simulink model "Klimaanlage_SIL"  (R2023b)
settings: Solver=FixedStepAuto  StartTime=0.0  StopTime=10.0  RelTol=1e-3
values from neighbouring files (symbols this model uses):
  T_a = 5    [qualification_test_01.m]    (also in qualification_test_02.m)
  T_i_start = 10    [qualification_test_01.m]    (also in qualification_test_02.m)
libraries: mbedblockslib x10, thermical_vehicelbody x1
settings Model: Creator=kilia  LastModifiedBy=kilia
settings HardwareCC: TargetBitPerPointer=64  TargetBitPerSizeT=64  TargetBitPerPtrDiffT=64  TargetLongLongMode=on  TargetIntDivRoundTo=Zero  TargetEndianess=LittleEndian  TargetWordSize=64  TargetHWDeviceType=MATLAB Host  ProdEqTarget=off
settings RTWCC: Description=S-Function Target  SystemTargetFile=rtwsfcn.tlc  TemplateMakefile=rtwsfcn_default_tmf
settings STFCustomTargetCC: ModelReferenceCompliant=off  CompOptLevelCompliant=on  MATLABClassNameForMDSCustomization=Simulink.SoftwareTarget.TargetSpecificTriggerConfigurationBase  GRTInterface=on  SystemTargetFile=rtwsfcn.tlc

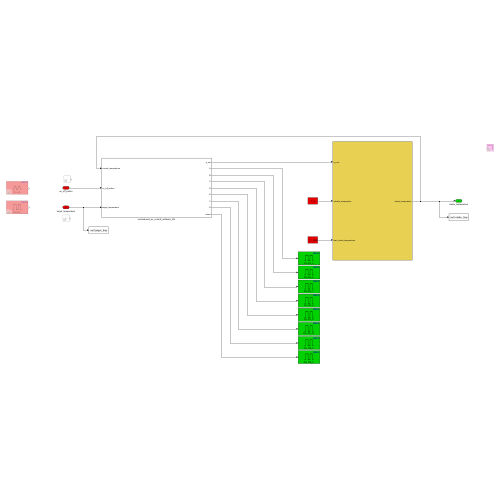
[thumbnail: Simulink's stored preview of the top-level diagram]
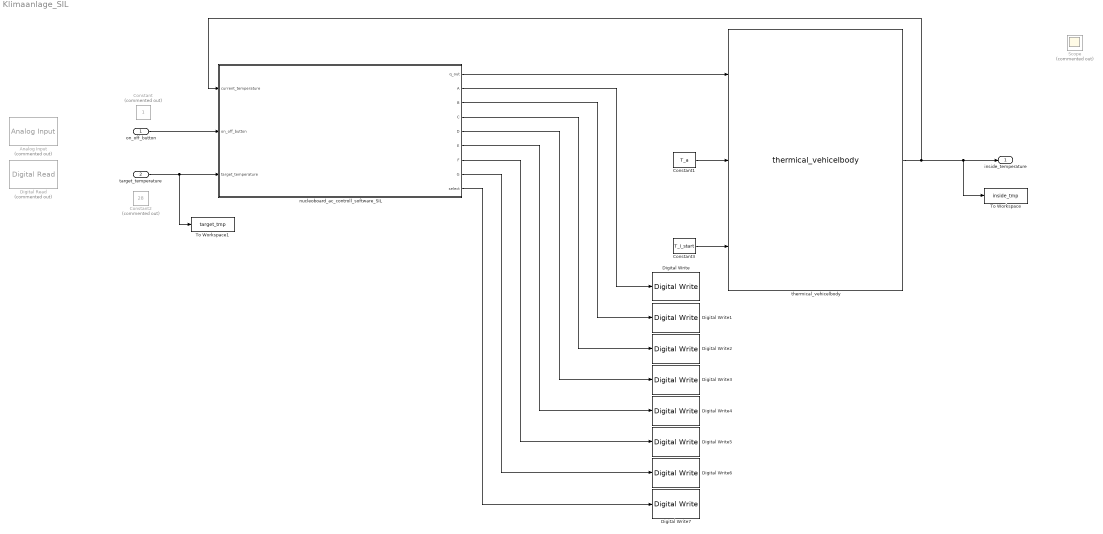
== system Klimaanlage_SIL ==
  on_off_button : Inport  OutDataTypeStr=boolean
  target_temperature : Inport  Port=2
  Analog Input : mbedblockslib/Analog Input  Commented=on  Pin=A0  ReadResultsOnly=off  ConversionTriggerSource=Software  ExternalTriggerType=uint32( 0 )  OutputDataType=double  EnableConversionCompleteNotify=off  EnableOuputStatus=off  SampleTime=-1
      settings: LibrarySourceBlock=stmnucleorootlib/Common/Analog Input
  Constant : Constant  Commented=on  OutDataTypeStr=boolean
  Constant1 : Constant  Value=T_a
  Constant2 : Constant  Commented=on  Value=28  OutDataTypeStr=uint16
  Constant3 : Constant  Value=T_i_start
  Digital Read : mbedblockslib/Digital Read  Commented=on  Pin=D2  Direction=input  SampleTime=-1
      settings: LibrarySourceBlock=stmnucleorootlib/Common/Digital Read
  Digital Write : mbedblockslib/Digital Write  Pin=PA_5  Direction=output
      settings: LibrarySourceBlock=stmnucleorootlib/Common/Digital Write
  Digital Write1 : mbedblockslib/Digital Write  Pin=PA_6  Direction=output
      settings: LibrarySourceBlock=stmnucleorootlib/Common/Digital Write
  Digital Write2 : mbedblockslib/Digital Write  Pin=PA_7  Direction=output
      settings: LibrarySourceBlock=stmnucleorootlib/Common/Digital Write
  Digital Write3 : mbedblockslib/Digital Write  Pin=PA_8  Direction=output
      settings: LibrarySourceBlock=stmnucleorootlib/Common/Digital Write
  Digital Write4 : mbedblockslib/Digital Write  Pin=PA_9  Direction=output
      settings: LibrarySourceBlock=stmnucleorootlib/Common/Digital Write
  Digital Write5 : mbedblockslib/Digital Write  Pin=PA_15  Direction=output
      settings: LibrarySourceBlock=stmnucleorootlib/Common/Digital Write
  Digital Write6 : mbedblockslib/Digital Write  Pin=PB_9  Direction=output
      settings: LibrarySourceBlock=stmnucleorootlib/Common/Digital Write
  Digital Write7 : mbedblockslib/Digital Write  Pin=PB_0  Direction=output
      settings: LibrarySourceBlock=stmnucleorootlib/Common/Digital Write
  Scope : Scope  Commented=on
  To Workspace : ToWorkspace  VariableName=inside_tmp  SaveFormat=Timeseries  SampleTime=-1
  To Workspace1 : ToWorkspace  VariableName=target_tmp  SaveFormat=Timeseries  SampleTime=-1
  nucleoboard_ac_controll_software_SIL : Subsystem
      mask help: Simulink:masks:GenSFuncDesc_MD
      mask Help: eval('feval(''rtwprivate'',''rtwhelpview'',''rtw_sfcn_block'')');
  thermical_vehicelbody : thermical_vehicelbody/thermical_vehicelbody  SystemSampleTime=-1  VariantActivationTime=update diagram  AllowFlexibleInterface=on  Latency=0  AutoFrameSizeCalculation=off
  inside_temperature : Outport
  wires:
  nucleoboard_ac_controll_software_SIL/8(G) -> Digital Write6/1
  nucleoboard_ac_controll_software_SIL/9(select) -> Digital Write7/1
  nucleoboard_ac_controll_software_SIL/6(E) -> Digital Write4/1
  Constant3/1 -> thermical_vehicelbody/3
  nucleoboard_ac_controll_software_SIL/3(B) -> Digital Write1/1
  nucleoboard_ac_controll_software_SIL/4(C) -> Digital Write2/1
  nucleoboard_ac_controll_software_SIL/7(F) -> Digital Write5/1
  nucleoboard_ac_controll_software_SIL/2(A) -> Digital Write/1
  nucleoboard_ac_controll_software_SIL/1(q_out) -> thermical_vehicelbody/1
  thermical_vehicelbody/1 -> To Workspace/1, inside_temperature/1, nucleoboard_ac_controll_software_SIL/1(current_temperature)
  Constant1/1 -> thermical_vehicelbody/2
  target_temperature/1 -> To Workspace1/1, nucleoboard_ac_controll_software_SIL/3(target_temperature)
  on_off_button/1 -> nucleoboard_ac_controll_software_SIL/2(on_off_button)
  nucleoboard_ac_controll_software_SIL/5(D) -> Digital Write3/1

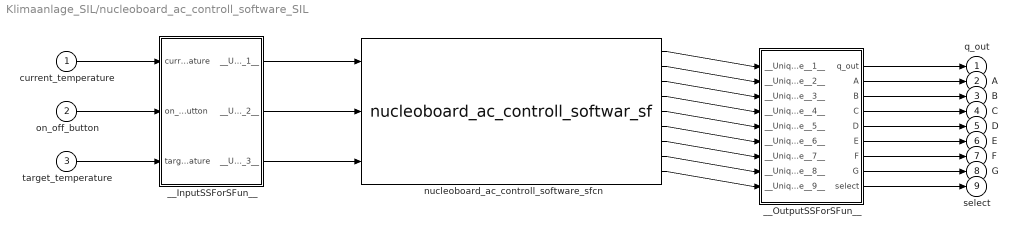
== system Klimaanlage_SIL/nucleoboard_ac_controll_software_SIL ==
  current_temperature : Inport
  on_off_button : Inport  Port=2
  target_temperature : Inport  Port=3
  __InputSSForSFun__ : Subsystem
  __OutputSSForSFun__ : Subsystem
  nucleoboard_ac_controll_software_sfcn : S-Function  FunctionName=nucleoboard_ac_controll_softwar_sf  SFunctionModules=""  SFunctionDeploymentMode=off  EnableBusSupport=off  SFcnStateName=DWORK0  mask{rtw_sf_name=nucleoboard_ac_controll_softwar_sf, showVar=off}
      mask prompts: rtw_sf_name "Simulink:masks:GenSFuncName_MP"; showVar "Simulink:masks:GenSFuncShowModuleList_MP"
      mask help: Simulink:masks:GenSFuncDesc_MD
      mask init:
      | displist = '';
      | if ~strcmp(get_param(gcb, 'FunctionName'), rtw_sf_name);
      |   set_param(gcb, 'FunctionName', rtw_sf_name);
      | end
      | % Check if we are generating code
      | rtw_mode = false;
      | if strcmpi(get_param(bdroot(gcb),'SimulationStatus'),'Initializing')
      | 	rtw_mode = strcmpi(get_param(bdroot(gcb),'BuildingRTWCode'),'on') && ...
      | 		~strcmpi(get_param(bdroot(gcb),'TargetStyle'),'SimulationTarget');
      | end
      | if showVar || rtw_mode
      | 	if exist('rtwsfunc') == 2 | exist('rtwsfunc') == 6
      | 		tmplist = rtwsfunc(rtw_sf_name,gcb);
      | 		tmplist = DAStudio.message('Simulink:masks:GenSFuncListOfModules_IC', tmplist);
      | 	elseif showVar
      | 		tmplist1 = DAStudio.message('Simulink:masks:GenSFuncListOfModules_IC', '');
      |         tmplist2 = DAStudio.message('Simulink:masks:GenSFuncNotLicensed_IC');
      |         tmplist = [tmplist1 tmplist2];
      |  	end
      | end
      | if showVar
      |   displist = tmplist;
      | end
      settings: SFcnIsStateOwnerBlock=on
      settings: CopyFcn=|
      | if ~strcmp(get_param(gcb,'Linkstatus'),'none') && ...
      | ~strcmp(get_param(gcb,'Linkstatus'),'implicit')
      |   set_param(gcb,'LinkStatus','none');
      | end
      mask Help: eval('feval(''rtwprivate'',''rtwhelpview'',''rtw_sfcn_block'')');
      mask Display:
      | port_label('input',1,'current_temperature');
      | port_label('input',2,'on_off_button');
      | port_label('input',3,'target_temperature');
      | port_label('output',1,'q_out');
      | port_label('output',2,'A');
      | port_label('output',3,'B');
      | port_label('output',4,'C');
      | port_label('output',5,'D');
      | port_label('output',6,'E');
      | port_label('output',7,'F');
      | port_label('output',8,'G');
      | port_label('output',9,'select');
  q_out : Outport
  A : Outport  Port=2
  B : Outport  Port=3
  C : Outport  Port=4
  D : Outport  Port=5
  E : Outport  Port=6
  F : Outport  Port=7
  G : Outport  Port=8
  select : Outport  Port=9
  wires:
  __OutputSSForSFun__/9(select) -> select/1
  __OutputSSForSFun__/8(G) -> G/1
  __OutputSSForSFun__/7(F) -> F/1
  __OutputSSForSFun__/6(E) -> E/1
  __OutputSSForSFun__/5(D) -> D/1
  __OutputSSForSFun__/4(C) -> C/1
  __OutputSSForSFun__/3(B) -> B/1
  __OutputSSForSFun__/2(A) -> A/1
  __OutputSSForSFun__/1(q_out) -> q_out/1
  nucleoboard_ac_controll_software_sfcn/9 -> __OutputSSForSFun__/9(__UniqueInportName__9__)
  nucleoboard_ac_controll_software_sfcn/8 -> __OutputSSForSFun__/8(__UniqueInportName__8__)
  nucleoboard_ac_controll_software_sfcn/7 -> __OutputSSForSFun__/7(__UniqueInportName__7__)
  nucleoboard_ac_controll_software_sfcn/6 -> __OutputSSForSFun__/6(__UniqueInportName__6__)
  nucleoboard_ac_controll_software_sfcn/5 -> __OutputSSForSFun__/5(__UniqueInportName__5__)
  nucleoboard_ac_controll_software_sfcn/4 -> __OutputSSForSFun__/4(__UniqueInportName__4__)
  nucleoboard_ac_controll_software_sfcn/3 -> __OutputSSForSFun__/3(__UniqueInportName__3__)
  nucleoboard_ac_controll_software_sfcn/2 -> __OutputSSForSFun__/2(__UniqueInportName__2__)
  nucleoboard_ac_controll_software_sfcn/1 -> __OutputSSForSFun__/1(__UniqueInportName__1__)
  __InputSSForSFun__/3(__UniqueOutportName__3__) -> nucleoboard_ac_controll_software_sfcn/3
  __InputSSForSFun__/2(__UniqueOutportName__2__) -> nucleoboard_ac_controll_software_sfcn/2
  __InputSSForSFun__/1(__UniqueOutportName__1__) -> nucleoboard_ac_controll_software_sfcn/1
  target_temperature/1 -> __InputSSForSFun__/3(target_temperature)
  on_off_button/1 -> __InputSSForSFun__/2(on_off_button)
  current_temperature/1 -> __InputSSForSFun__/1(current_temperature)

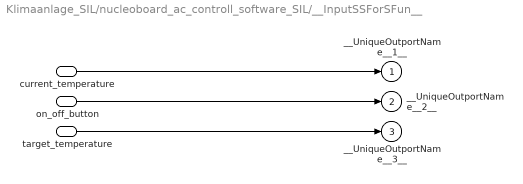
== system Klimaanlage_SIL/nucleoboard_ac_controll_software_SIL/__InputSSForSFun__ ==
  current_temperature : Inport
  on_off_button : Inport  Port=2
  target_temperature : Inport  Port=3
  __UniqueOutportName__1__ : Outport
  __UniqueOutportName__2__ : Outport  Port=2
  __UniqueOutportName__3__ : Outport  Port=3
  wires:
  target_temperature/1 -> __UniqueOutportName__3__/1
  on_off_button/1 -> __UniqueOutportName__2__/1
  current_temperature/1 -> __UniqueOutportName__1__/1

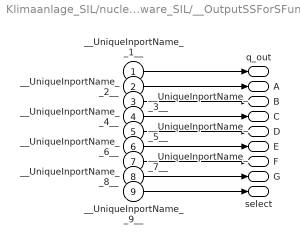
== system Klimaanlage_SIL/nucleoboard_ac_controll_software_SIL/__OutputSSForSFun__ ==
  __UniqueInportName__1__ : Inport
  __UniqueInportName__2__ : Inport  Port=2
  __UniqueInportName__3__ : Inport  Port=3
  __UniqueInportName__4__ : Inport  Port=4
  __UniqueInportName__5__ : Inport  Port=5
  __UniqueInportName__6__ : Inport  Port=6
  __UniqueInportName__7__ : Inport  Port=7
  __UniqueInportName__8__ : Inport  Port=8
  __UniqueInportName__9__ : Inport  Port=9
  q_out : Outport
  A : Outport  Port=2
  B : Outport  Port=3
  C : Outport  Port=4
  D : Outport  Port=5
  E : Outport  Port=6
  F : Outport  Port=7
  G : Outport  Port=8
  select : Outport  Port=9
  wires:
  __UniqueInportName__9__/1 -> select/1
  __UniqueInportName__8__/1 -> G/1
  __UniqueInportName__7__/1 -> F/1
  __UniqueInportName__6__/1 -> E/1
  __UniqueInportName__5__/1 -> D/1
  __UniqueInportName__4__/1 -> C/1
  __UniqueInportName__3__/1 -> B/1
  __UniqueInportName__2__/1 -> A/1
  __UniqueInportName__1__/1 -> q_out/1
